simulink model "sensing"  (R2020a)
settings: Solver=FixedStepAuto  StartTime=0.0  StopTime=10.0  FixedStep=1e-3  RelTol=1e-3  EnableMultiTasking=on
settings Model: ExtModeTrigDuration=5  Creator=zhanz173  LastModifiedBy=zhanz173
settings OptimizationCC: EnhancedBackFolding=on  PassReuseOutputArgsAs=Individual arguments  ZeroExternalMemoryAtStartup=off  ZeroInternalMemoryAtStartup=off  MaxStackSize=64  OptimizeBlockOrder=speed  DifferentSizesBufferReuse=on  OptimizationCustomize=off  EfficientTunableParamExpr=on
settings DebuggingCC: ParameterTunabilityLossMsg=error
settings HardwareCC: ProdBitPerPointer=32  ProdBitPerSizeT=32  ProdBitPerPtrDiffT=32  ProdLargestAtomicInteger=Long  ProdLargestAtomicFloat=Double  ProdWordSize=32  ProdHWDeviceType=ARM Compatible->ARM Cortex  TargetBitPerPointer=64  TargetBitPerSizeT=64  TargetBitPerPtrDiffT=64  TargetLongLongMode=on  TargetIntDivRoundTo=Zero  TargetEndianess=LittleEndian  TargetWordSize=64  TargetHWDeviceType=Custom Processor->MATLAB Host Computer  ProdEqTarget=off
settings SFSimCC: MATLABDynamicMemAlloc=off
settings RTWCC: SystemTargetFile=ert.tlc  HardwareBoard=NXP FRDM-K64F  TemplateMakefile=ert_default_tmf  Toolchain=GNU Tools for ARM Embedded Processors
settings CodeAppCC: ForceParamTrailComments=on  IgnoreCustomStorageClasses=off  OperatorAnnotations=on  SimulinkDataObjDesc=on  SFDataObjDesc=on  InsertBlockDesc=on

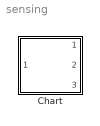
== system sensing ==
  Chart : Stateflow chart  TreatAsAtomicUnit=on

== stateflow chart sensing/Chart ==
  state IDLE
    entry:
  state stage2
    entry:
    ATR_CMP_REF_PWM = 1
    FRONTEND_CTRL = 1
  state stage3
    entry:
    VENT_CMP_REF_PWM = 1
    FRONTEND_CTRL = 1
  state RESET
    entry:
    ATR_CMP_REF_PWM = 0
    VENT_CMP_REF_PWM = 0
    FRONTEND_CTRL = 0
  RESET -> IDLE
  (default) -> IDLE
  IDLE -> stage2 [order 1] : [mode == 3]
  IDLE -> stage3 [order 2] : [mode == 4]
  stage2 -> RESET
  stage3 -> RESET
  data: ATR_CMP_REF_PWM output; VENT_CMP_REF_PWM output; FRONTEND_CTRL output; mode input
